simulink model "mod_5_count"  (R2020a)
settings: Solver=VariableStepAuto  StartTime=0.0  StopTime=inf  RelTol=1e-3
settings Model: Creator=Shubham  LastModifiedBy=Shubham

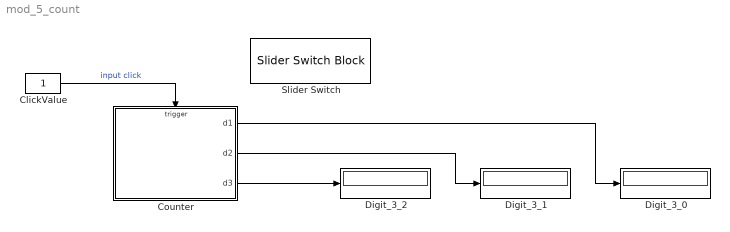
== system mod_5_count ==
  ClickValue : Constant
  Counter : Stateflow chart  TreatAsAtomicUnit=on
  Digit_3_0 : Display
  Digit_3_1 : Display
  Digit_3_2 : Display
  Slider Switch : SliderSwitchBlock  LabelPosition=Bottom
      settings: Values={{'Off', 'On'}, [0 1]}
  wires:
  ClickValue/1 -> Counter/Trigger  "input click"
  Counter/3(d3) -> Digit_3_2/1
  Counter/2(d2) -> Digit_3_1/1
  Counter/1(d1) -> Digit_3_0/1

== stateflow chart mod_5_count/Counter ==
  settings: executeAtInitialization=1
  state digit1 [parallel]
    settings: executionOrder=1
    state one
      en: d1 = 1;
    state two
      en: d1 = 2;
    state zero
      en: d1 = 0;
    digit1.zero -> digit1.one : inputClick
    digit1.one -> digit1.two : inputClick
    (default) -> digit1.zero
    digit1.two -> digit1.zero : inputClick /{digit2.inc2;}
  state digit2 [parallel]
    settings: executionOrder=2
    state one
      en: d2 = 1;
    state two
      en: d2 = 2;
    state zero
      en: d2 = 0;
    digit2.zero -> digit2.one : inc2
    digit2.one -> digit2.two : inc2
    (default) -> digit2.zero
    digit2.two -> digit2.zero : inc2 /{digit3.inc3;}
  state digit3 [parallel]
    settings: executionOrder=3
    state one
      en: d3 = 1;
    state two
      en: d3 = 2;
    state zero
      en: d3 = 0;
    digit3.zero -> digit3.one : inc3
    digit3.one -> digit3.two : inc3
    (default) -> digit3.zero
    digit3.two -> digit3.zero : inc3
  data: d1 output size=1; d2 output size=1; d3 output size=1
  events: inc2 local EITHER_EDGE_EVENT; inc3 local EITHER_EDGE_EVENT; inputClick input EITHER_EDGE_EVENT
